simulink subsystem "TCS"  (R2025b)
settings: Solver=VariableStepAuto  StartTime=0.0  StopTime=10.0  RelTol=1e-3
settings Model: Creator=mjmag  LastModifiedBy=diego
settings RTWCC: GPUComputeCapability=3.5

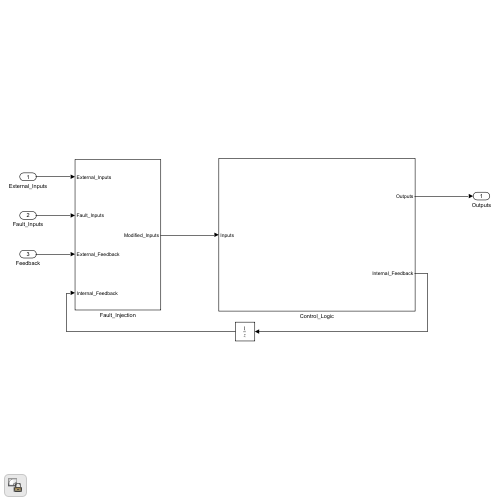
[thumbnail: Simulink's stored preview of the top-level diagram]
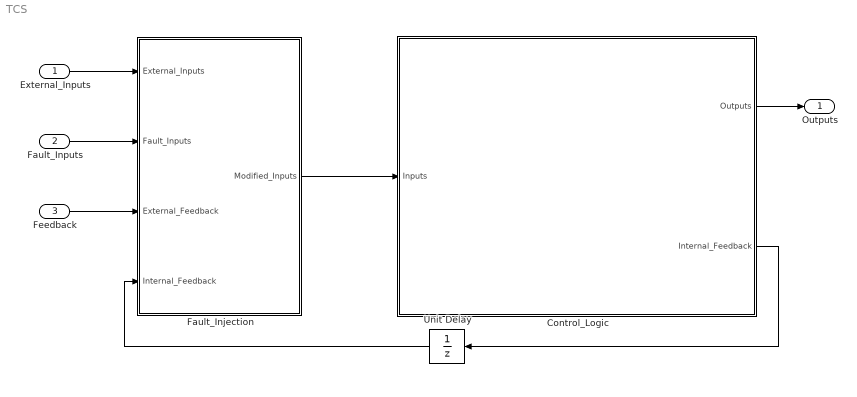
== system TCS ==
  External_Inputs : Inport
  Fault_Inputs : Inport  Port=2
  Feedback : Inport  Port=3
  Control_Logic : Subsystem
  Fault_Injection : Subsystem
  Unit Delay : UnitDelay  SampleTime=-1  HasFrameUpgradeWarning=on
  Outputs : Outport
  wires:
  Fault_Injection/1(Modified_Inputs) -> Control_Logic/1(Inputs)
  Fault_Inputs/1 -> Fault_Injection/2(Fault_Inputs)
  Control_Logic/2(Internal_Feedback) -> Unit Delay/1
  External_Inputs/1 -> Fault_Injection/1(External_Inputs)
  Feedback/1 -> Fault_Injection/3(External_Feedback)
  Unit Delay/1 -> Fault_Injection/4(Internal_Feedback)
  Control_Logic/1(Outputs) -> Outputs/1

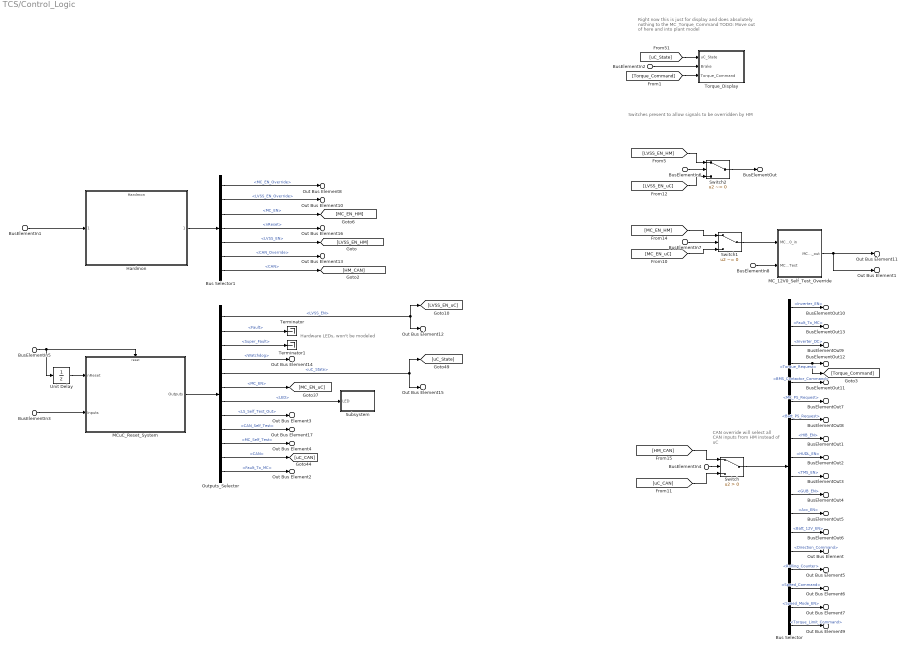
== system TCS/Control_Logic ==
  note: Right now this is just for display and does absolutely nothing to the MC_Torque_Command
      |
      | TODO: Move out of here and into plant model
  note: Switches present to allow signals
      | to be overridden by HM
  note: CAN override will select all CAN inputs from HM instead of uC
  note: Hardware LEDs, won't be modeled
  BusElementIn3 : Inport  PortName=Inputs
  BusElementIn1 : Inport  PortName=Inputs
  BusElementIn2 : Inport  PortName=Inputs  Element=Rider_Inputs.Brake
  BusElementIn4 : Inport  PortName=Inputs  Element=Feedback.Internal_Feedback.CAN_Override
  BusElementIn5 : Inport  PortName=Inputs  Element=Feedback.Internal_Feedback.nReset
  BusElementIn6 : Inport  PortName=Inputs  Element=Feedback.Internal_Feedback.LVSS_EN_Override
  BusElementIn7 : Inport  PortName=Inputs  Element=Feedback.Internal_Feedback.MC_EN_Override
  BusElementIn8 : Inport  PortName=Inputs  Element=Feedback.Internal_Feedback.MC_Self_Test
  Bus Selector : BusSelector  OutputSignals=Inverter_EN,Fault_To_MC,Inverter_DC,Torque_Request,BMS_Contactor_Command,MC_PS_Request,Batt_PS_Request,HIB_EN,HUDL_EN,TMS_EN,GUB_EN,Acc_EN,Batt_12V_EN,Direction_Command,Rolling_Counter,Speed_Command,Speed_Mode_EN,Torque_Limit_Command
  Bus Selector1 : BusSelector  OutputSignals=MC_EN_Override,LVSS_EN_Override,MC_EN,nReset,LVSS_EN,CAN_Override,CAN
  Hardmon : ModelReference  ModelNameDialog=Hardmon  SimulationMode=Normal  ModelReferenceVersion=1.106
  MC_12V0_Self_Test_Override : Subsystem
  "MCuC_Reset_System " : Subsystem  TreatAsAtomicUnit=on
  Outputs_Selector : BusSelector  OutputSignals=LVSS_EN,Fault,Super_Fault,Watchdog,uC_State,MC_EN,LED,LS_Self_Test_Out,CAN_Self_Test,MC_Self_Test,CAN,CAN.Fault_To_MC
  Subsystem : Subsystem
  Switch : Switch  Criteria=u2 > Threshold  OutDataTypeStr=Inherit: Inherit via back propagation  SaturateOnIntegerOverflow=off  InputSameDT=off
  Switch1 : Switch  Criteria=u2 ~= 0  SaturateOnIntegerOverflow=off  InputSameDT=off
  Switch2 : Switch  Criteria=u2 ~= 0  SaturateOnIntegerOverflow=off  InputSameDT=off
  Terminator : Terminator
  Terminator1 : Terminator
  Torque_Display : Subsystem
  Unit Delay : UnitDelay  SampleTime=-1  HasFrameUpgradeWarning=on
  Out Bus Element : Outport  PortName=Outputs  Element=MC_Outputs.MC_Command.Direction_Command
  Out Bus Element5 : Outport  PortName=Outputs  Element=MC_Outputs.MC_Command.Rolling_Counter
  Out Bus Element6 : Outport  PortName=Outputs  Element=MC_Outputs.MC_Command.Speed_Command
  Out Bus Element7 : Outport  PortName=Outputs  Element=MC_Outputs.MC_Command.Speed_Mode_Enable
  Out Bus Element9 : Outport  PortName=Outputs  Element=MC_Outputs.MC_Command.Torque_Limit_Command
  Out Bus Element2 : Outport  PortName=Outputs  Element=MC_Outputs.Fault_To_MC
  Out Bus Element1 : Outport  PortName=Outputs  Element=MC_Outputs.MC_12V0
  BusElementOut1 : Outport  PortName=Outputs  Element=LVSS_Outputs.HIB_EN
  BusElementOut2 : Outport  PortName=Outputs  Element=LVSS_Outputs.HUDL_EN
  BusElementOut3 : Outport  PortName=Outputs  Element=LVSS_Outputs.TMS_EN
  BusElementOut4 : Outport  PortName=Outputs  Element=LVSS_Outputs.GUB_EN
  BusElementOut5 : Outport  PortName=Outputs  Element=LVSS_Outputs.Acc_EN
  BusElementOut6 : Outport  PortName=Outputs  Element=LVSS_Outputs.Batt_12V_EN
  BusElementOut7 : Outport  PortName=Outputs  Element=TMS_Outputs.MC_Speed
  BusElementOut8 : Outport  PortName=Outputs  Element=TMS_Outputs.Batt_Speed
  BusElementOut9 : Outport  PortName=Outputs  Element=VCU_Outputs.Inverter_Discharge
  BusElementOut10 : Outport  PortName=Outputs  Element=VCU_Outputs.Inverter_Enable
  BusElementOut11 : Outport  PortName=Outputs  Element=VCU_Outputs.BMS_Contactor_Command
  BusElementOut12 : Outport  PortName=Outputs  Element=VCU_Outputs.Torque_Command
  BusElementOut13 : Outport  PortName=Outputs  Element=VCU_Outputs.Fault_To_MC
  BusElementOut : Outport  PortName=Outputs  Element=LVSS_Output.LSS_EN
  Out Bus Element12 : Outport  Port=2  PortName=Internal_Feedback  Element=LVSS_EN
  Out Bus Element14 : Outport  Port=2  PortName=Internal_Feedback  Element=Watchdog
  Out Bus Element15 : Outport  Port=2  PortName=Internal_Feedback  Element=uC_State
  Out Bus Element17 : Outport  Port=2  PortName=Internal_Feedback  Element=CAN_Self_Test
  Out Bus Element11 : Outport  Port=2  PortName=Internal_Feedback  Element=MC_12V0
  Out Bus Element3 : Outport  Port=2  PortName=Internal_Feedback  Element=LS_Self_Test
  Out Bus Element4 : Outport  Port=2  PortName=Internal_Feedback  Element=MC_Self_Test
  Out Bus Element8 : Outport  Port=2  PortName=Internal_Feedback  Element=MC_EN_Override
  Out Bus Element10 : Outport  Port=2  PortName=Internal_Feedback  Element=LVSS_EN_Override
  Out Bus Element13 : Outport  Port=2  PortName=Internal_Feedback  Element=CAN_Override
  Out Bus Element16 : Outport  Port=2  PortName=Internal_Feedback  Element=nReset
  wires:
  Bus Selector/18 -> Out Bus Element9/1  "<Torque_Limit_Command>"
  Bus Selector/17 -> Out Bus Element7/1  "<Speed_Mode_EN>"
  Bus Selector/16 -> Out Bus Element6/1  "<Speed_Command>"
  Bus Selector/15 -> Out Bus Element5/1  "<Rolling_Counter>"
  Bus Selector/14 -> Out Bus Element/1  "<Direction_Command>"
  Bus Selector/13 -> BusElementOut6/1  "<Batt_12V_EN>"
  Bus Selector/12 -> BusElementOut5/1  "<Acc_EN>"
  Bus Selector/11 -> BusElementOut4/1  "<GUB_EN>"
  Bus Selector/10 -> BusElementOut3/1  "<TMS_EN>"
  Bus Selector/9 -> BusElementOut2/1  "<HUDL_EN>"
  Bus Selector/8 -> BusElementOut1/1  "<HIB_EN>"
  Bus Selector/7 -> BusElementOut8/1  "<Batt_PS_Request>"
  Bus Selector/6 -> BusElementOut7/1  "<MC_PS_Request>"
  Bus Selector/5 -> BusElementOut11/1  "<BMS_Contactor_Command>"
  [Torque_Command] -> Torque_Display/3(Torque_Command)
  Bus Selector/4 -> BusElementOut12/1, [Torque_Command]  "<Torque_Request>"
  Bus Selector/3 -> BusElementOut9/1  "<Inverter_DC>"
  Bus Selector/2 -> BusElementOut13/1  "<Fault_To_MC>"
  Bus Selector/1 -> BusElementOut10/1  "<Inverter_EN>"
  Bus Selector1/7 -> [HM_CAN]  "<CAN>"
  Bus Selector1/6 -> Out Bus Element13/1  "<CAN_Override>"
  Bus Selector1/5 -> [LVSS_EN_HM]  "<LVSS_EN>"
  Bus Selector1/4 -> Out Bus Element16/1  "<nReset>"
  Bus Selector1/3 -> [MC_EN_HM]  "<MC_EN>"
  Bus Selector1/2 -> Out Bus Element10/1  "<LVSS_EN_Override>"
  Bus Selector1/1 -> Out Bus Element8/1  "<MC_EN_Override>"
  Hardmon/1 -> Bus Selector1/1
  BusElementIn1/1 -> Hardmon/1
  Outputs_Selector/11 -> [uC_CAN]  "<CAN>"
  Outputs_Selector/12 -> Out Bus Element2/1  "<Fault_To_MC>"
  Outputs_Selector/3 -> Terminator1/1  "<Super_Fault>"
  Outputs_Selector/2 -> Terminator/1  "<Fault>"
  Outputs_Selector/10 -> Out Bus Element4/1  "<MC_Self_Test>"
  Outputs_Selector/8 -> Out Bus Element3/1  "<LS_Self_Test_Out>"
  "MCuC_Reset_System "/1(Outputs) -> Outputs_Selector/1
  BusElementIn3/1 -> "MCuC_Reset_System "/2(Inputs)
  Outputs_Selector/5 -> [uC_State], Out Bus Element15/1  "<uC_State>"
  Outputs_Selector/4 -> Out Bus Element14/1  "<Watchdog>"
  Outputs_Selector/1 -> [LVSS_EN_uC], Out Bus Element12/1  "<LVSS_EN>"
  Outputs_Selector/7 -> Subsystem/1(LED)  "<LED>"
  Outputs_Selector/9 -> Out Bus Element17/1  "<CAN_Self_Test>"
  Outputs_Selector/6 -> [MC_EN_uC]  "<MC_EN>"
  [HM_CAN] -> Switch/1
  [LVSS_EN_HM] -> Switch2/1
  Switch2/1 -> BusElementOut/1
  BusElementIn6/1 -> Switch2/2
  [LVSS_EN_uC] -> Switch2/3
  BusElementIn8/1 -> MC_12V0_Self_Test_Override/2(MC_Self_Test)
  MC_12V0_Self_Test_Override/1(MC_12V0_out) -> Out Bus Element1/1, Out Bus Element11/1
  [MC_EN_HM] -> Switch1/1
  BusElementIn7/1 -> Switch1/2
  Switch1/1 -> MC_12V0_Self_Test_Override/1(MC_12V0_in)
  [MC_EN_uC] -> Switch1/3
  BusElementIn5/1 -> "MCuC_Reset_System "/Reset, Unit Delay/1
  Switch/1 -> Bus Selector/1
  [uC_CAN] -> Switch/3
  BusElementIn4/1 -> Switch/2
  Unit Delay/1 -> "MCuC_Reset_System "/1(nReset)
  [uC_State] -> Torque_Display/1(uC_State)
  BusElementIn2/1 -> Torque_Display/2(Brake)

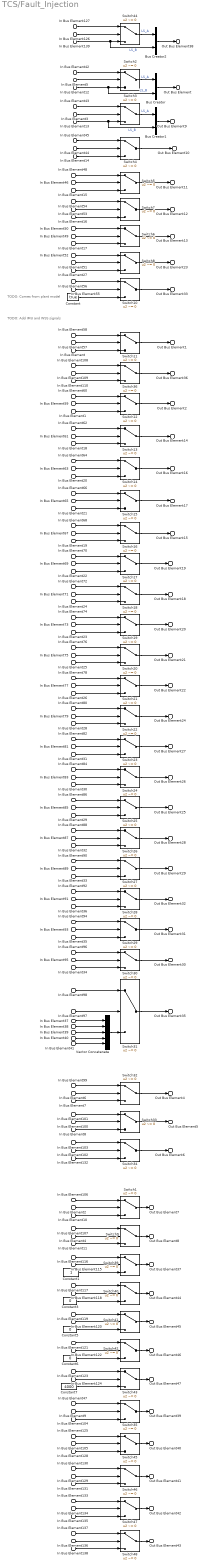
== system TCS/Fault_Injection ==
  note: TODO: Add IMU and WSS signals
  note: TODO: Comes from plant model
  In Bus Element12 : Inport  PortName=External_Inputs  Element=No_HIB.Key_In
  In Bus Element13 : Inport  PortName=External_Inputs  Element=No_HIB.Estop_In
  In Bus Element17 : Inport  PortName=External_Inputs  Element=Yes_HIB.Throttle
  In Bus Element16 : Inport  PortName=External_Inputs  Element=Yes_HIB.Start
  In Bus Element15 : Inport  PortName=External_Inputs  Element=Yes_HIB.Forward_EN
  In Bus Element14 : Inport  PortName=External_Inputs  Element=Yes_HIB.Brake
  In Bus Element27 : Inport  PortName=External_Inputs  Element=Yes_HIB.HIB_Comparison_Fault
  In Bus Element41 : Inport  PortName=External_Inputs  Element=Yes_HIB.HIB_Heartbeat
  In Bus Element2 : Inport  Port=2  PortName=Fault_Inputs  Element=Override_Watchdog
  In Bus Element3 : Inport  Port=2  PortName=Fault_Inputs  Element=Override_Back_Wheel_Speed
  In Bus Element4 : Inport  Port=2  PortName=Fault_Inputs  Element=Override_uC_State
  In Bus Element5 : Inport  Port=2  PortName=Fault_Inputs  Element=Override_Front_Wheel_Speed
  In Bus Element42 : Inport  Port=2  PortName=Fault_Inputs  Element=Front_Wheel_Speed
  In Bus Element43 : Inport  Port=2  PortName=Fault_Inputs  Element=Back_Wheel_Speed
  In Bus Element44 : Inport  Port=2  PortName=Fault_Inputs  Element=Override_Brake
  In Bus Element45 : Inport  Port=2  PortName=Fault_Inputs  Element=Brake
  In Bus Element46 : Inport  Port=2  PortName=Fault_Inputs  Element=Override_Forward_EN
  In Bus Element48 : Inport  Port=2  PortName=Fault_Inputs  Element=Forward_EN
  In Bus Element53 : Inport  Port=2  PortName=Fault_Inputs  Element=Override_Start
  In Bus Element54 : Inport  Port=2  PortName=Fault_Inputs  Element=Start
  In Bus Element50 : Inport  Port=2  PortName=Fault_Inputs  Element=Throttle
  In Bus Element49 : Inport  Port=2  PortName=Fault_Inputs  Element=Override_Throttle
  In Bus Element51 : Inport  Port=2  PortName=Fault_Inputs  Element=Override_HIB_Comparison_Fault
  In Bus Element52 : Inport  Port=2  PortName=Fault_Inputs  Element=HIB_Comparison_Fault
  In Bus Element56 : Inport  Port=2  PortName=Fault_Inputs  Element=Interlock
  In Bus Element55 : Inport  Port=2  PortName=Fault_Inputs  Element=Override_Interlock
  In Bus Element59 : Inport  Port=2  PortName=Fault_Inputs  Element=Override_LVSS_ON
  In Bus Element60 : Inport  Port=2  PortName=Fault_Inputs  Element=LVSS_ON
  In Bus Element61 : Inport  Port=2  PortName=Fault_Inputs  Element=Override_Contactor_Closed
  In Bus Element62 : Inport  Port=2  PortName=Fault_Inputs  Element=Contactor_Closed
  In Bus Element63 : Inport  Port=2  PortName=Fault_Inputs  Element=Override_Cell_Temps
  In Bus Element64 : Inport  Port=2  PortName=Fault_Inputs  Element=Cell_Temps
  In Bus Element65 : Inport  Port=2  PortName=Fault_Inputs  Element=Override_Cell_Voltages
  In Bus Element66 : Inport  Port=2  PortName=Fault_Inputs  Element=Cell_Voltages
  In Bus Element67 : Inport  Port=2  PortName=Fault_Inputs  Element=Override_Isolation_State
  In Bus Element68 : Inport  Port=2  PortName=Fault_Inputs  Element=Isolation_State
  In Bus Element69 : Inport  Port=2  PortName=Fault_Inputs  Element=Override_MC_Speed_Out
  In Bus Element70 : Inport  Port=2  PortName=Fault_Inputs  Element=MC_Speed_Out
  In Bus Element71 : Inport  Port=2  PortName=Fault_Inputs  Element=Override_Batt_Speed_Out
  In Bus Element72 : Inport  Port=2  PortName=Fault_Inputs  Element=Batt_Speed_Out
  In Bus Element73 : Inport  Port=2  PortName=Fault_Inputs  Element=Override_Temperatures
  In Bus Element74 : Inport  Port=2  PortName=Fault_Inputs  Element=Temperatures
  In Bus Element75 : Inport  Port=2  PortName=Fault_Inputs  Element=Override_MC_Flow_Rate
  In Bus Element76 : Inport  Port=2  PortName=Fault_Inputs  Element=MC_Flow_Rate
  In Bus Element77 : Inport  Port=2  PortName=Fault_Inputs  Element=Override_Batt_Flow_Rate
  In Bus Element78 : Inport  Port=2  PortName=Fault_Inputs  Element=Batt_Flow_Rate
  In Bus Element79 : Inport  Port=2  PortName=Fault_Inputs  Element=Override_HIB_ON
  In Bus Element80 : Inport  Port=2  PortName=Fault_Inputs  Element=HIB_ON
  In Bus Element81 : Inport  Port=2  PortName=Fault_Inputs  Element=Override_HUDL_ON
  In Bus Element82 : Inport  Port=2  PortName=Fault_Inputs  Element=HUDL_ON
  In Bus Element83 : Inport  Port=2  PortName=Fault_Inputs  Element=Override_TMS_ON
  In Bus Element84 : Inport  Port=2  PortName=Fault_Inputs  Element=TMS_ON
  In Bus Element85 : Inport  Port=2  PortName=Fault_Inputs  Element=Override_GUB_ON
  In Bus Element86 : Inport  Port=2  PortName=Fault_Inputs  Element=GUB_ON
  In Bus Element87 : Inport  Port=2  PortName=Fault_Inputs  Element=Override_Acc_ON
  In Bus Element88 : Inport  Port=2  PortName=Fault_Inputs  Element=Acc_ON
  In Bus Element89 : Inport  Port=2  PortName=Fault_Inputs  Element=Override_Batt_12V_ON
  In Bus Element90 : Inport  Port=2  PortName=Fault_Inputs  Element=Batt_12V_ON
  In Bus Element91 : Inport  Port=2  PortName=Fault_Inputs  Element=Override_Vicor_Current
  In Bus Element92 : Inport  Port=2  PortName=Fault_Inputs  Element=Vicor_Current
  In Bus Element93 : Inport  Port=2  PortName=Fault_Inputs  Element=Override_LVSS_Temps
  In Bus Element94 : Inport  Port=2  PortName=Fault_Inputs  Element=LVSS_Temps
  In Bus Element95 : Inport  Port=2  PortName=Fault_Inputs  Element=Override_LVSS_Currents
  In Bus Element96 : Inport  Port=2  PortName=Fault_Inputs  Element=LVSS_Currents
  In Bus Element97 : Inport  Port=2  PortName=Fault_Inputs  Element=Override_Heartbeats
  In Bus Element98 : Inport  Port=2  PortName=Fault_Inputs  Element=Heartbeats
  In Bus Element6 : Inport  Port=2  PortName=Fault_Inputs  Element=Override_MC_12V0
  In Bus Element99 : Inport  Port=2  PortName=Fault_Inputs  Element=MC_12V0
  In Bus Element100 : Inport  Port=2  PortName=Fault_Inputs  Element=Override_LVSS_EN
  In Bus Element101 : Inport  Port=2  PortName=Fault_Inputs  Element=LVSS_EN
  In Bus Element102 : Inport  Port=2  PortName=Fault_Inputs  Element=Override_nReset
  In Bus Element103 : Inport  Port=2  PortName=Fault_Inputs  Element=nReset
  In Bus Element106 : Inport  Port=2  PortName=Fault_Inputs  Element=Watchdog
  In Bus Element107 : Inport  Port=2  PortName=Fault_Inputs  Element=uC_State
  In Bus Element57 : Inport  Port=2  PortName=Fault_Inputs  Element=Override_Inverter_Discharge_State
  In Bus Element58 : Inport  Port=2  PortName=Fault_Inputs  Element=Inverter_Discharge_State
  In Bus Element109 : Inport  Port=2  PortName=Fault_Inputs  Element=Override_VSM_State
  In Bus Element108 : Inport  Port=2  PortName=Fault_Inputs  Element=VSM_State
  In Bus Element116 : Inport  Port=2  PortName=Fault_Inputs  Element=Direction_Command
  In Bus Element115 : Inport  Port=2  PortName=Fault_Inputs  Element=Override_Direction_Command
  In Bus Element117 : Inport  Port=2  PortName=Fault_Inputs  Element=Rolling_Counter
  In Bus Element118 : Inport  Port=2  PortName=Fault_Inputs  Element=Override_Rolling_Counter
  In Bus Element119 : Inport  Port=2  PortName=Fault_Inputs  Element=Speed_Command
  In Bus Element120 : Inport  Port=2  PortName=Fault_Inputs  Element=Override_Speed_Command
  In Bus Element121 : Inport  Port=2  PortName=Fault_Inputs  Element=Speed_Mode_Enable
  In Bus Element122 : Inport  Port=2  PortName=Fault_Inputs  Element=Override_Speed_Mode_Enable
  In Bus Element123 : Inport  Port=2  PortName=Fault_Inputs  Element=Torque_Limit_Command
  In Bus Element124 : Inport  Port=2  PortName=Fault_Inputs  Element=Override_Torque_Limit_Command
  In Bus Element127 : Inport  Port=2  PortName=Fault_Inputs  Element=LS_Self_Test
  In Bus Element126 : Inport  Port=2  PortName=Fault_Inputs  Element=Override_LS_Self_Test
  In Bus Element9 : Inport  Port=2  PortName=Fault_Inputs  Element=Override_CAN_Override
  In Bus Element47 : Inport  Port=2  PortName=Fault_Inputs  Element=CAN_Override
  In Bus Element125 : Inport  Port=2  PortName=Fault_Inputs  Element=LVSS_EN_Override
  In Bus Element105 : Inport  Port=2  PortName=Fault_Inputs  Element=Override_LVSS_EN_Override
  In Bus Element130 : Inport  Port=2  PortName=Fault_Inputs  Element=MC_EN_Override
  In Bus Element129 : Inport  Port=2  PortName=Fault_Inputs  Element=Override_MC_EN_Override
  In Bus Element133 : Inport  Port=2  PortName=Fault_Inputs  Element=MC_Self_Test
  In Bus Element134 : Inport  Port=2  PortName=Fault_Inputs  Element=Override_MC_Self_Test
  In Bus Element137 : Inport  Port=2  PortName=Fault_Inputs  Element=CAN_Self_Test
  In Bus Element136 : Inport  Port=2  PortName=Fault_Inputs  Element=Override_CAN_Self_Test
  In Bus Element : Inport  Port=3  PortName=External_Feedback  Element=MC_Feedback.D4_Inverter_Discharge_State
  In Bus Element110 : Inport  Port=3  PortName=External_Feedback  Element=MC_Feedback.D1_VSM_State
  In Bus Element28 : Inport  Port=3  PortName=External_Feedback  Element=LVSS_Feedback.HIB_ON
  In Bus Element1 : Inport  Port=3  PortName=External_Feedback  Element=LVSS_Feedback.LVSS_ON
  In Bus Element31 : Inport  Port=3  PortName=External_Feedback  Element=LVSS_Feedback.HUDL_ON
  In Bus Element30 : Inport  Port=3  PortName=External_Feedback  Element=LVSS_Feedback.TMS_ON
  In Bus Element29 : Inport  Port=3  PortName=External_Feedback  Element=LVSS_Feedback.GUB_ON
  In Bus Element32 : Inport  Port=3  PortName=External_Feedback  Element=LVSS_Feedback.Acc_ON
  In Bus Element33 : Inport  Port=3  PortName=External_Feedback  Element=LVSS_Feedback.Batt_12V_ON
  In Bus Element36 : Inport  Port=3  PortName=External_Feedback  Element=LVSS_Feedback.Vicor_Current
  In Bus Element35 : Inport  Port=3  PortName=External_Feedback  Element=LVSS_Feedback.LVSS_Temps
  In Bus Element34 : Inport  Port=3  PortName=External_Feedback  Element=LVSS_Feedback.LVSS_Currents
  In Bus Element37 : Inport  Port=3  PortName=External_Feedback  Element=LVSS_Feedback.LVSS_Heartbeat
  In Bus Element18 : Inport  Port=3  PortName=External_Feedback  Element=BMS_Feedback.BMS_Feedback.Contactor_Closed
  In Bus Element20 : Inport  Port=3  PortName=External_Feedback  Element=BMS_Feedback.BMS_Feedback.Cell_Temps
  In Bus Element21 : Inport  Port=3  PortName=External_Feedback  Element=BMS_Feedback.BMS_Feedback.Cell_Voltages
  In Bus Element39 : Inport  Port=3  PortName=External_Feedback  Element=BMS_Feedback.BMS_Feedback.BMS_Heartbeat
  In Bus Element19 : Inport  Port=3  PortName=External_Feedback  Element=GFDB_Feedback.GFDB_Feedback.Isolation_State
  In Bus Element40 : Inport  Port=3  PortName=External_Feedback  Element=GFDB_Feedback.GFDB_Feedback.GFDB_Heartbeat
  In Bus Element22 : Inport  Port=3  PortName=External_Feedback  Element=TMS_Feedback.MC_Speed_Out
  In Bus Element24 : Inport  Port=3  PortName=External_Feedback  Element=TMS_Feedback.Batt_Speed_Out
  In Bus Element23 : Inport  Port=3  PortName=External_Feedback  Element=TMS_Feedback.Temperatures
  In Bus Element25 : Inport  Port=3  PortName=External_Feedback  Element=TMS_Feedback.MC_Flow_Rate
  In Bus Element26 : Inport  Port=3  PortName=External_Feedback  Element=TMS_Feedback.Batt_Flow_Rate
  In Bus Element38 : Inport  Port=3  PortName=External_Feedback  Element=TMS_Feedback.TMS_Heartbeat
  In Bus Element7 : Inport  Port=4  PortName=Internal_Feedback  Element=MC_12V0
  In Bus Element8 : Inport  Port=4  PortName=Internal_Feedback  Element=LVSS_EN
  In Bus Element10 : Inport  Port=4  PortName=Internal_Feedback  Element=Watchdog
  In Bus Element11 : Inport  Port=4  PortName=Internal_Feedback  Element=uC_State
  In Bus Element104 : Inport  Port=4  PortName=Internal_Feedback  Element=CAN_Override
  In Bus Element128 : Inport  Port=4  PortName=Internal_Feedback  Element=LVSS_EN_Override
  In Bus Element131 : Inport  Port=4  PortName=Internal_Feedback  Element=MC_EN_Override
  In Bus Element132 : Inport  Port=4  PortName=Internal_Feedback  Element=nReset
  In Bus Element135 : Inport  Port=4  PortName=Internal_Feedback  Element=MC_Self_Test
  In Bus Element138 : Inport  Port=4  PortName=Internal_Feedback  Element=CAN_Self_Test
  In Bus Element139 : Inport  Port=4  PortName=Internal_Feedback  Element=LS_Self_Test
  Bus Creator : BusCreator  Inputs=2
  Bus Creator1 : BusCreator  Inputs=2
  Bus Creator2 : BusCreator  Inputs=2
  Constant : Constant  Value=true
  Constant1 : Constant
  Constant3 : Constant  Value=0
  Constant5 : Constant  Value=0
  Constant6 : Constant  Value=0
  Constant7 : Constant  Value=4000
  Switch{1..36,39..48} (46 alike) : Switch  Criteria=u2 ~= 0  OutDataTypeStr=Inherit: Inherit via back propagation  SaturateOnIntegerOverflow=off  InputSameDT=off
  Vector Concatenate : Concatenate  NumInputs=5
  Out Bus Element : Outport  PortName=Modified_Inputs  Element=Rider_Inputs.Key_In
  Out Bus Element9 : Outport  PortName=Modified_Inputs  Element=Rider_Inputs.Estop_In
  Out Bus Element10 : Outport  PortName=Modified_Inputs  Element=Rider_Inputs.Brake
  Out Bus Element11 : Outport  PortName=Modified_Inputs  Element=Rider_Inputs.Forward_EN
  Out Bus Element12 : Outport  PortName=Modified_Inputs  Element=Rider_Inputs.Start
  Out Bus Element13 : Outport  PortName=Modified_Inputs  Element=Rider_Inputs.Throttle
  Out Bus Element1 : Outport  PortName=Modified_Inputs  Element=Feedback.MC_Feedback.D4_Inverter_Discharge_State
  Out Bus Element36 : Outport  PortName=Modified_Inputs  Element=Feedback.MC_Feedback.D1_VSM_State
  Out Bus Element2 : Outport  PortName=Modified_Inputs  Element=Feedback.LVSS_Feedback.LVSS_ON
  Out Bus Element24 : Outport  PortName=Modified_Inputs  Element=Feedback.LVSS_Feedback.HIB_ON
  Out Bus Element25 : Outport  PortName=Modified_Inputs  Element=Feedback.LVSS_Feedback.GUB_ON
  Out Bus Element26 : Outport  PortName=Modified_Inputs  Element=Feedback.LVSS_Feedback.TMS_ON
  Out Bus Element27 : Outport  PortName=Modified_Inputs  Element=Feedback.LVSS_Feedback.HUDL_ON
  Out Bus Element28 : Outport  PortName=Modified_Inputs  Element=Feedback.LVSS_Feedback.Acc_ON
  Out Bus Element29 : Outport  PortName=Modified_Inputs  Element=Feedback.LVSS_Feedback.Batt_12V_ON
  Out Bus Element30 : Outport  PortName=Modified_Inputs  Element=Feedback.LVSS_Feedback.LVSS_Currents
  Out Bus Element31 : Outport  PortName=Modified_Inputs  Element=Feedback.LVSS_Feedback.LVSS_Temps
  Out Bus Element32 : Outport  PortName=Modified_Inputs  Element=Feedback.LVSS_Feedback.Vicor_Current
  Out Bus Element4 : Outport  PortName=Modified_Inputs  Element=Feedback.Internal_Feedback.MC_12V0
  Out Bus Element5 : Outport  PortName=Modified_Inputs  Element=Feedback.Internal_Feedback.LVSS_EN_uC
  Out Bus Element6 : Outport  PortName=Modified_Inputs  Element=Feedback.Internal_Feedback.nReset
  Out Bus Element7 : Outport  PortName=Modified_Inputs  Element=Feedback.Internal_Feedback.Watchdog
  Out Bus Element8 : Outport  PortName=Modified_Inputs  Element=Feedback.Internal_Feedback.uC_State
  Out Bus Element39 : Outport  PortName=Modified_Inputs  Element=Feedback.Internal_Feedback.CAN_Override
  Out Bus Element40 : Outport  PortName=Modified_Inputs  Element=Feedback.Internal_Feedback.LVSS_EN_Override
  Out Bus Element41 : Outport  PortName=Modified_Inputs  Element=Feedback.Internal_Feedback.MC_EN_Override
  Out Bus Element42 : Outport  PortName=Modified_Inputs  Element=Feedback.Internal_Feedback.MC_Self_Test
  Out Bus Element43 : Outport  PortName=Modified_Inputs  Element=Feedback.Internal_Feedback.CAN_Self_Test
  Out Bus Element14 : Outport  PortName=Modified_Inputs  Element=Feedback.BMS_Feedback.Contactor_Closed
  Out Bus Element16 : Outport  PortName=Modified_Inputs  Element=Feedback.BMS_Feedback.Cell_Temps
  Out Bus Element17 : Outport  PortName=Modified_Inputs  Element=Feedback.BMS_Feedback.Cell_Voltages
  Out Bus Element15 : Outport  PortName=Modified_Inputs  Element=Feedback.GFDB_Feedback.Isolation_State
  Out Bus Element19 : Outport  PortName=Modified_Inputs  Element=Feedback.TMS_Feedback.MC_Speed_Out
  Out Bus Element18 : Outport  PortName=Modified_Inputs  Element=Feedback.TMS_Feedback.Batt_Speed_Out
  Out Bus Element20 : Outport  PortName=Modified_Inputs  Element=Feedback.TMS_Feedback.Temperatures
  Out Bus Element21 : Outport  PortName=Modified_Inputs  Element=Feedback.TMS_Feedback.MC_Flow_Rate
  Out Bus Element22 : Outport  PortName=Modified_Inputs  Element=Feedback.TMS_Feedback.Batt_Flow_Rate
  Out Bus Element35 : Outport  PortName=Modified_Inputs  Element=Feedback.Heartbeats
  Out Bus Element23 : Outport  PortName=Modified_Inputs  Element=HIB.HIB_Comparison_Fault
  Out Bus Element33 : Outport  PortName=Modified_Inputs  Element=Interlock
  Out Bus Element37 : Outport  PortName=Modified_Inputs  Element=MC_Direction_Command
  Out Bus Element44 : Outport  PortName=Modified_Inputs  Element=MC_Rolling_Counter
  Out Bus Element45 : Outport  PortName=Modified_Inputs  Element=MC_Speed_Command
  Out Bus Element46 : Outport  PortName=Modified_Inputs  Element=MC_Speed_Mode_Enable
  Out Bus Element47 : Outport  PortName=Modified_Inputs  Element=MC_Torque_Limit_Command
  Out Bus Element38 : Outport  PortName=Modified_Inputs  Element=Internal_Feedback.LS_Self_Test
  wires:
  In Bus Element138/1 -> Switch48/3
  In Bus Element136/1 -> Switch48/2
  In Bus Element137/1 -> Switch48/1
  Switch48/1 -> Out Bus Element43/1
  Switch47/1 -> Out Bus Element42/1
  In Bus Element133/1 -> Switch47/1
  In Bus Element134/1 -> Switch47/2
  In Bus Element135/1 -> Switch47/3
  In Bus Element131/1 -> Switch46/3
  In Bus Element129/1 -> Switch46/2
  In Bus Element130/1 -> Switch46/1
  Switch46/1 -> Out Bus Element41/1
  Switch45/1 -> Out Bus Element40/1
  In Bus Element125/1 -> Switch45/1
  In Bus Element105/1 -> Switch45/2
  In Bus Element128/1 -> Switch45/3
  In Bus Element104/1 -> Switch35/3
  In Bus Element9/1 -> Switch35/2
  In Bus Element47/1 -> Switch35/1
  Switch35/1 -> Out Bus Element39/1
  In Bus Element132/1 -> Switch34/3
  In Bus Element139/1 -> Switch44/3, Bus Creator2/2  "LS_B"
  In Bus Element126/1 -> Switch44/2
  Switch44/1 -> Bus Creator2/1  "LS_A"
  Bus Creator2/1 -> Out Bus Element38/1
  In Bus Element127/1 -> Switch44/1
  Constant7/1 -> Switch43/3
  Constant6/1 -> Switch42/3
  Constant5/1 -> Switch41/3
  Constant3/1 -> Switch40/3
  Constant1/1 -> Switch39/3
  In Bus Element124/1 -> Switch43/2
  In Bus Element123/1 -> Switch43/1
  In Bus Element122/1 -> Switch42/2
  In Bus Element121/1 -> Switch42/1
  In Bus Element120/1 -> Switch41/2
  In Bus Element119/1 -> Switch41/1
  In Bus Element118/1 -> Switch40/2
  In Bus Element117/1 -> Switch40/1
  In Bus Element115/1 -> Switch39/2
  In Bus Element116/1 -> Switch39/1
  Switch43/1 -> Out Bus Element47/1
  Switch42/1 -> Out Bus Element46/1
  Switch41/1 -> Out Bus Element45/1
  Switch40/1 -> Out Bus Element44/1
  Switch39/1 -> Out Bus Element37/1
  In Bus Element108/1 -> Switch36/1
  In Bus Element110/1 -> Switch36/3
  Switch36/1 -> Out Bus Element36/1
  In Bus Element109/1 -> Switch36/2
  In Bus Element41/1 -> Vector Concatenate/5
  In Bus Element40/1 -> Vector Concatenate/4
  In Bus Element37/1 -> Vector Concatenate/1
  In Bus Element38/1 -> Vector Concatenate/2
  In Bus Element39/1 -> Vector Concatenate/3
  In Bus Element13/1 -> Switch3/3, Bus Creator1/2  "LS_B"
  Bus Creator1/1 -> Out Bus Element9/1
  In Bus Element43/1 -> Switch3/1
  Switch3/1 -> Bus Creator1/1  "LS_A"
  In Bus Element3/1 -> Switch3/2
  In Bus Element5/1 -> Switch2/2
  Switch2/1 -> Bus Creator/1  "LS_A"
  In Bus Element42/1 -> Switch2/1
  Bus Creator/1 -> Out Bus Element/1
  In Bus Element12/1 -> Switch2/3, Bus Creator/2  "LS_B"
  In Bus Element2/1 -> Switch1/2
  Switch1/1 -> Out Bus Element7/1
  In Bus Element106/1 -> Switch1/1
  Switch9/1 -> Out Bus Element8/1
  In Bus Element107/1 -> Switch9/1
  In Bus Element4/1 -> Switch9/2
  In Bus Element11/1 -> Switch9/3
  In Bus Element10/1 -> Switch1/3
  In Bus Element44/1 -> Switch4/2
  In Bus Element45/1 -> Switch4/1
  In Bus Element14/1 -> Switch4/3
  Switch4/1 -> Out Bus Element10/1
  Switch5/1 -> Out Bus Element11/1
  In Bus Element15/1 -> Switch5/3
  In Bus Element46/1 -> Switch5/2
  In Bus Element48/1 -> Switch5/1
  Switch7/1 -> Out Bus Element12/1
  In Bus Element53/1 -> Switch7/2
  In Bus Element54/1 -> Switch7/1
  In Bus Element16/1 -> Switch7/3
  In Bus Element49/1 -> Switch6/2
  In Bus Element50/1 -> Switch6/1
  Switch6/1 -> Out Bus Element13/1
  In Bus Element17/1 -> Switch6/3
  In Bus Element51/1 -> Switch8/2
  In Bus Element52/1 -> Switch8/1
  Switch8/1 -> Out Bus Element23/1
  In Bus Element27/1 -> Switch8/3
  In Bus Element55/1 -> Switch10/2
  In Bus Element56/1 -> Switch10/1
  Switch10/1 -> Out Bus Element33/1
  Constant/1 -> Switch10/3
  In Bus Element57/1 -> Switch11/2
  In Bus Element58/1 -> Switch11/1
  Switch11/1 -> Out Bus Element1/1
  In Bus Element/1 -> Switch11/3
  In Bus Element59/1 -> Switch12/2
  In Bus Element60/1 -> Switch12/1
  Switch12/1 -> Out Bus Element2/1
  In Bus Element1/1 -> Switch12/3
  In Bus Element61/1 -> Switch13/2
  In Bus Element62/1 -> Switch13/1
  Switch13/1 -> Out Bus Element14/1
  In Bus Element18/1 -> Switch13/3
  In Bus Element63/1 -> Switch14/2
  In Bus Element64/1 -> Switch14/1
  Switch14/1 -> Out Bus Element16/1
  In Bus Element20/1 -> Switch14/3
  In Bus Element65/1 -> Switch15/2
  In Bus Element66/1 -> Switch15/1
  Switch15/1 -> Out Bus Element17/1
  In Bus Element21/1 -> Switch15/3
  In Bus Element67/1 -> Switch16/2
  In Bus Element68/1 -> Switch16/1
  Switch16/1 -> Out Bus Element15/1
  In Bus Element19/1 -> Switch16/3
  In Bus Element69/1 -> Switch17/2
  In Bus Element70/1 -> Switch17/1
  Switch17/1 -> Out Bus Element19/1
  In Bus Element22/1 -> Switch17/3
  In Bus Element71/1 -> Switch18/2
  In Bus Element72/1 -> Switch18/1
  Switch18/1 -> Out Bus Element18/1
  In Bus Element24/1 -> Switch18/3
  In Bus Element73/1 -> Switch19/2
  In Bus Element74/1 -> Switch19/1
  Switch19/1 -> Out Bus Element20/1
  In Bus Element23/1 -> Switch19/3
  In Bus Element75/1 -> Switch20/2
  In Bus Element76/1 -> Switch20/1
  Switch20/1 -> Out Bus Element21/1
  In Bus Element25/1 -> Switch20/3
  In Bus Element77/1 -> Switch21/2
  In Bus Element78/1 -> Switch21/1
  Switch21/1 -> Out Bus Element22/1
  In Bus Element26/1 -> Switch21/3
  In Bus Element79/1 -> Switch22/2
  In Bus Element80/1 -> Switch22/1
  Switch22/1 -> Out Bus Element24/1
  In Bus Element28/1 -> Switch22/3
  In Bus Element81/1 -> Switch23/2
  In Bus Element82/1 -> Switch23/1
  Switch23/1 -> Out Bus Element27/1
  In Bus Element31/1 -> Switch23/3
  In Bus Element83/1 -> Switch24/2
  In Bus Element84/1 -> Switch24/1
  Switch24/1 -> Out Bus Element26/1
  In Bus Element30/1 -> Switch24/3
  In Bus Element85/1 -> Switch25/2
  In Bus Element86/1 -> Switch25/1
  Switch25/1 -> Out Bus Element25/1
  In Bus Element29/1 -> Switch25/3
  In Bus Element87/1 -> Switch26/2
  In Bus Element88/1 -> Switch26/1
  Switch26/1 -> Out Bus Element28/1
  In Bus Element32/1 -> Switch26/3
  In Bus Element89/1 -> Switch27/2
  In Bus Element90/1 -> Switch27/1
  Switch27/1 -> Out Bus Element29/1
  In Bus Element33/1 -> Switch27/3
  In Bus Element91/1 -> Switch28/2
  In Bus Element92/1 -> Switch28/1
  Switch28/1 -> Out Bus Element32/1
  In Bus Element36/1 -> Switch28/3
  In Bus Element93/1 -> Switch29/2
  In Bus Element94/1 -> Switch29/1
  Switch29/1 -> Out Bus Element31/1
  In Bus Element35/1 -> Switch29/3
  In Bus Element95/1 -> Switch30/2
  In Bus Element96/1 -> Switch30/1
  Switch30/1 -> Out Bus Element30/1
  In Bus Element34/1 -> Switch30/3
  In Bus Element97/1 -> Switch31/2
  In Bus Element98/1 -> Switch31/1
  Switch31/1 -> Out Bus Element35/1
  Vector Concatenate/1 -> Switch31/3
  In Bus Element6/1 -> Switch32/2
  In Bus Element7/1 -> Switch32/3
  In Bus Element99/1 -> Switch32/1
  Switch32/1 -> Out Bus Element4/1
  In Bus Element100/1 -> Switch33/2
  In Bus Element8/1 -> Switch33/3
  In Bus Element101/1 -> Switch33/1
  Switch33/1 -> Out Bus Element5/1
  In Bus Element102/1 -> Switch34/2
  In Bus Element103/1 -> Switch34/1
  Switch34/1 -> Out Bus Element6/1

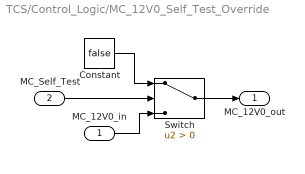
== system TCS/Control_Logic/MC_12V0_Self_Test_Override ==
  MC_12V0_in : Inport
  MC_Self_Test : Inport  Port=2
  Constant : Constant  Value=false
  Switch : Switch  Criteria=u2 > Threshold  SaturateOnIntegerOverflow=off  InputSameDT=off
  MC_12V0_out : Outport
  wires:
  MC_12V0_in/1 -> Switch/3
  Constant/1 -> Switch/1
  Switch/1 -> MC_12V0_out/1
  MC_Self_Test/1 -> Switch/2

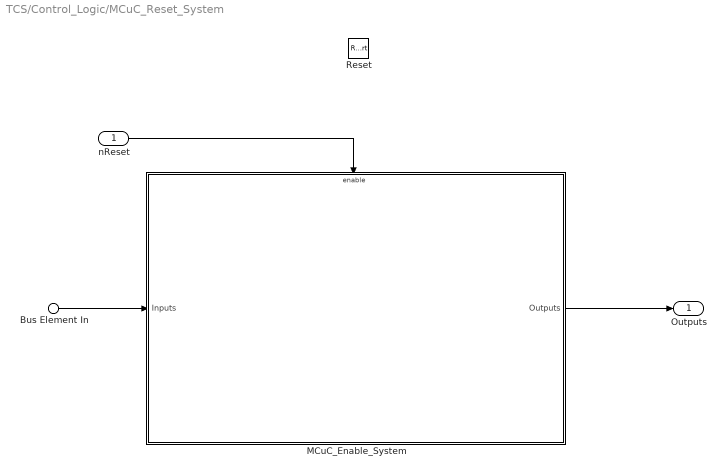
== system TCS/Control_Logic/MCuC_Reset_System  ==
  nReset : Inport
  Bus Element In : Inport  Port=2  PortName=Inputs
  Reset : ResetPort  DisableCoverage=on
  "MCuC_Enable_System " : Subsystem  TreatAsAtomicUnit=on
  Outputs : Outport
  wires:
  "MCuC_Enable_System "/1(Outputs) -> Outputs/1
  Bus Element In/1 -> "MCuC_Enable_System "/1(Inputs)
  nReset/1 -> "MCuC_Enable_System "/Enable

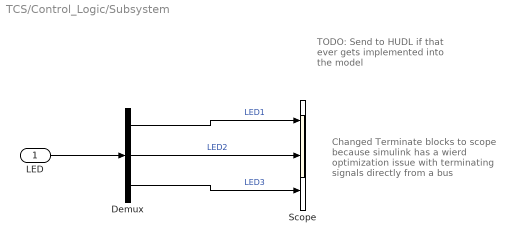
== system TCS/Control_Logic/Subsystem ==
  note: Changed Terminate blocks to scope because simulink has a wierd optimization issue with terminating signals directly from a bus
  note: TODO: Send to HUDL if that ever gets implemented into the model
  LED : Inport  PortDimensions=[1 3]
  Demux : Demux  Outputs=3
  Scope : Scope  NumInputPorts=3
  wires:
  Demux/3 -> Scope/3  "LED3"
  Demux/1 -> Scope/1  "LED1"
  Demux/2 -> Scope/2  "LED2"
  LED/1 -> Demux/1

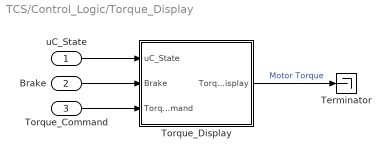
== system TCS/Control_Logic/Torque_Display ==
  uC_State : Inport
  Brake : Inport  Port=2
  Torque_Command : Inport  Port=3
  Terminator : Terminator
  Torque_Display : Stateflow chart  TreatAsAtomicUnit=on
  wires:
  Torque_Display/1(Torque_Display) -> Terminator/1  "Motor Torque"
  Brake/1 -> Torque_Display/2(Brake)
  Torque_Command/1 -> Torque_Display/3(Torque_Command)
  uC_State/1 -> Torque_Display/1(uC_State)

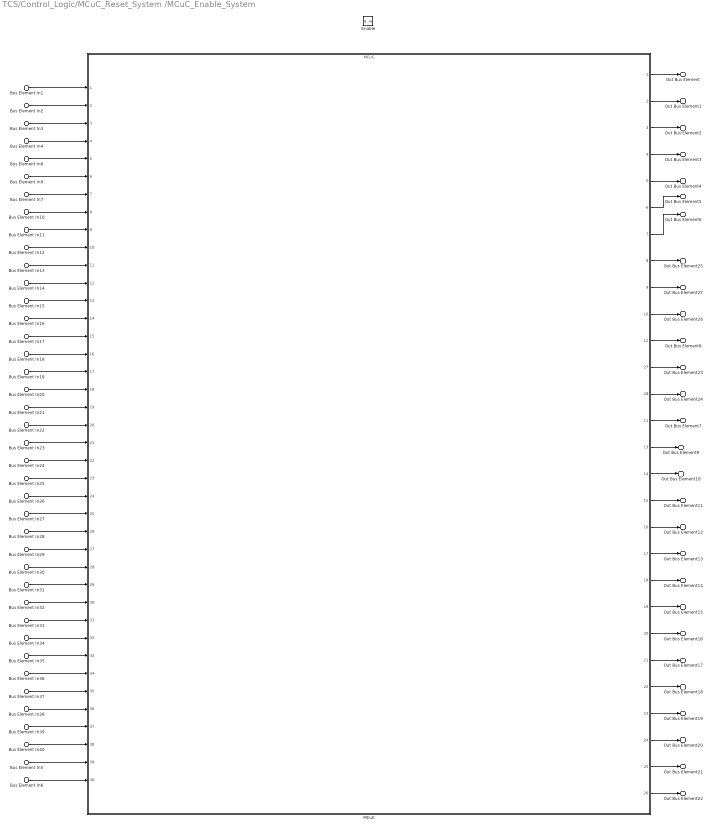
== system TCS/Control_Logic/MCuC_Reset_System /MCuC_Enable_System  ==
  Bus Element In1 : Inport  PortName=Inputs  Element=Rider_Inputs.Key_In.LS_A
  Bus Element In2 : Inport  PortName=Inputs  Element=Rider_Inputs.Key_In.LS_B
  Bus Element In3 : Inport  PortName=Inputs  Element=Rider_Inputs.Estop_In.LS_A
  Bus Element In4 : Inport  PortName=Inputs  Element=Rider_Inputs.Estop_In.LS_B
  Bus Element In9 : Inport  PortName=Inputs  Element=Rider_Inputs.Start
  Bus Element In11 : Inport  PortName=Inputs  Element=Rider_Inputs.Brake
  Bus Element In12 : Inport  PortName=Inputs  Element=Rider_Inputs.Forward_EN
  Bus Element In15 : Inport  PortName=Inputs  Element=Rider_Inputs.Throttle
  Bus Element In5 : Inport  PortName=Inputs  Element=Internal_Feedback.LS_Self_Test.LS_A
  Bus Element In6 : Inport  PortName=Inputs  Element=Internal_Feedback.LS_Self_Test.LS_B
  Bus Element In7 : Inport  PortName=Inputs  Element=Interlock
  Bus Element In8 : Inport  PortName=Inputs  Element=Feedback.Internal_Feedback.MC_12V0
  Bus Element In10 : Inport  PortName=Inputs  Element=Feedback.LVSS_Feedback.LVSS_ON
  Bus Element In26 : Inport  PortName=Inputs  Element=Feedback.LVSS_Feedback.HIB_ON
  Bus Element In27 : Inport  PortName=Inputs  Element=Feedback.LVSS_Feedback.HUDL_ON
  Bus Element In28 : Inport  PortName=Inputs  Element=Feedback.LVSS_Feedback.TMS_ON
  Bus Element In29 : Inport  PortName=Inputs  Element=Feedback.LVSS_Feedback.GUB_ON
  Bus Element In30 : Inport  PortName=Inputs  Element=Feedback.LVSS_Feedback.Acc_ON
  Bus Element In31 : Inport  PortName=Inputs  Element=Feedback.LVSS_Feedback.Batt_12V_ON
  Bus Element In32 : Inport  PortName=Inputs  Element=Feedback.LVSS_Feedback.Vicor_Current
  Bus Element In33 : Inport  PortName=Inputs  Element=Feedback.LVSS_Feedback.LVSS_Temps
  Bus Element In34 : Inport  PortName=Inputs  Element=Feedback.LVSS_Feedback.LVSS_Currents
  Bus Element In13 : Inport  PortName=Inputs  Element=Feedback.MC_Feedback.D1_VSM_State
  Bus Element In14 : Inport  PortName=Inputs  Element=Feedback.MC_Feedback.D4_Inverter_Discharge_State
  Bus Element In16 : Inport  PortName=Inputs  Element=Feedback.BMS_Feedback.Contactor_Closed
  Bus Element In17 : Inport  PortName=Inputs  Element=Feedback.BMS_Feedback.Cell_Temps
  Bus Element In18 : Inport  PortName=Inputs  Element=Feedback.BMS_Feedback.Cell_Voltages
  Bus Element In19 : Inport  PortName=Inputs  Element=Feedback.GFDB_Feedback.Isolation_State
  Bus Element In20 : Inport  PortName=Inputs  Element=Feedback.TMS_Feedback.MC_Speed_Out
  Bus Element In21 : Inport  PortName=Inputs  Element=Feedback.TMS_Feedback.Batt_Speed_Out
  Bus Element In22 : Inport  PortName=Inputs  Element=Feedback.TMS_Feedback.Temperatures
  Bus Element In23 : Inport  PortName=Inputs  Element=Feedback.TMS_Feedback.MC_Flow_Rate
  Bus Element In24 : Inport  PortName=Inputs  Element=Feedback.TMS_Feedback.Batt_Flow_Rate
  Bus Element In35 : Inport  PortName=Inputs  Element=Feedback.Heartbeats
  Bus Element In25 : Inport  PortName=Inputs  Element=HIB.HIB_Comparison_Fault
  Bus Element In36 : Inport  PortName=Inputs  Element=MC_Direction_Command
  Bus Element In37 : Inport  PortName=Inputs  Element=MC_Rolling_Counter
  Bus Element In38 : Inport  PortName=Inputs  Element=MC_Speed_Command
  Bus Element In39 : Inport  PortName=Inputs  Element=MC_Speed_Mode_Enable
  Bus Element In40 : Inport  PortName=Inputs  Element=MC_Torque_Limit_Command
  Enable : EnablePort
  MCuC : ModelReference  ModelNameDialog=MCuC.slx  SimulationMode=Normal  ModelReferenceVersion=5.3
      settings: PortSchema="{\"entries\":[{\"content\":{\"sides\":[{\"content\":{\"connectorIds\":[\"In1\",\"In2\",\"In3\",\"In4\",\"In5\",\"In6\",\"In7\",\"In8\",\"In9\",\"In10\",\"In11\",\"In12\",\"In13\",\"In14\",\"In15\",\"In16\",\"In17\",\"In18\",\"In19\",\"In20\",\"In21\",\"In22\",\"In23\",\"In24\",\"In25\",\"In26\",\"In27\",\"In28\",\"In29\",\"In30\",\"In31\",\"In32\",\"In33\",\"In34\",\"In35\",\"In36\",\"In37\",\"In38\",\"In39\",\"In40\"]},\"type\":\"ConnectorPlacement.EquallySpacedRectSide\",\"uuid\":\"380f24c8-28c2-4d84-ada4-76c3689d45f6\"},{\"content\":{\"connectorIds\":[\"Out1\",\"Out2\",\"Out3\",\"Out4\",\"Out5\",\"Out6\",\"Out7\",\"Out8\",\"Out9\",\"Out10\",\"Out12\",\"Out27\",\"Out28\",\"Out11\",\"Out13\",\"Out14\",\"Out15\",\"Out16\",\"Out17\",\"Out18\",\"Out19\",\"Out20\",\"Out21\",\"Out22\",\"Out23\",\"Out24\",\"Out25\",\"Out26\"],\"side\":\"RIGHT\"},\"type\":\"ConnectorPlacement.EquallySpacedRectSide\",\"uuid\":\"ebd1e0cb-fd96-46a4-b253-2ab002a0179d\"},{\"content\":{\"side\":\"TOP\"},\"type\":\"ConnectorPlacement.EquallySpacedRectSide\",\"uuid\":\"2c6ccd3c-3f8f-4b48-bb10-6601e3a9f937\"}]},\"type\":\"ConnectorPlacement.EquallySpacedConnector\",\"uuid\":\"9fb03b06-08d2-4f18-a55b-57581e35a7b0\"}],\"packageUris\":[\"http://schema.mathworks.com/mf0/Connector/R2020b\"],\"version\":\"1.0\"}"
  Out Bus Element : Outport  PortName=Outputs  Element=LVSS_EN
  Out Bus Element1 : Outport  PortName=Outputs  Element=Fault
  Out Bus Element2 : Outport  PortName=Outputs  Element=Super_Fault
  Out Bus Element3 : Outport  PortName=Outputs  Element=Watchdog
  Out Bus Element4 : Outport  PortName=Outputs  Element=uC_State
  Out Bus Element5 : Outport  PortName=Outputs  Element=MC_EN
  Out Bus Element6 : Outport  PortName=Outputs  Element=LED
  Out Bus Element7 : Outport  PortName=Outputs  Element=CAN.Inverter_EN
  Out Bus Element8 : Outport  PortName=Outputs  Element=CAN.Fault_To_MC
  Out Bus Element9 : Outport  PortName=Outputs  Element=CAN.Inverter_DC
  Out Bus Element10 : Outport  PortName=Outputs  Element=CAN.Torque_Request
  Out Bus Element11 : Outport  PortName=Outputs  Element=CAN.BMS_Contactor_Command
  Out Bus Element12 : Outport  PortName=Outputs  Element=CAN.MC_PS_Request
  Out Bus Element13 : Outport  PortName=Outputs  Element=CAN.Batt_PS_Request
  Out Bus Element14 : Outport  PortName=Outputs  Element=CAN.HIB_EN
  Out Bus Element15 : Outport  PortName=Outputs  Element=CAN.HUDL_EN
  Out Bus Element16 : Outport  PortName=Outputs  Element=CAN.TMS_EN
  Out Bus Element17 : Outport  PortName=Outputs  Element=CAN.GUB_EN
  Out Bus Element18 : Outport  PortName=Outputs  Element=CAN.Acc_EN
  Out Bus Element19 : Outport  PortName=Outputs  Element=CAN.Batt_12V_EN
  Out Bus Element20 : Outport  PortName=Outputs  Element=CAN.Direction_Command
  Out Bus Element21 : Outport  PortName=Outputs  Element=CAN.Rolling_Counter
  Out Bus Element22 : Outport  PortName=Outputs  Element=CAN.Speed_Command
  Out Bus Element23 : Outport  PortName=Outputs  Element=CAN.Speed_Mode_EN
  Out Bus Element24 : Outport  PortName=Outputs  Element=CAN.Torque_Limit_Command
  Out Bus Element25 : Outport  PortName=Outputs  Element=LS_Self_Test_Out
  Out Bus Element27 : Outport  PortName=Outputs  Element=CAN_Self_Test
  Out Bus Element26 : Outport  PortName=Outputs  Element=MC_Self_Test
  wires:
  MCuC/26 -> Out Bus Element22/1
  MCuC/25 -> Out Bus Element21/1
  MCuC/24 -> Out Bus Element20/1
  MCuC/23 -> Out Bus Element19/1
  MCuC/22 -> Out Bus Element18/1
  MCuC/21 -> Out Bus Element17/1
  MCuC/20 -> Out Bus Element16/1
  MCuC/19 -> Out Bus Element15/1
  MCuC/18 -> Out Bus Element14/1
  MCuC/17 -> Out Bus Element13/1
  MCuC/16 -> Out Bus Element12/1
  MCuC/15 -> Out Bus Element11/1
  MCuC/14 -> Out Bus Element10/1
  MCuC/13 -> Out Bus Element9/1
  MCuC/11 -> Out Bus Element7/1
  MCuC/28 -> Out Bus Element24/1
  MCuC/27 -> Out Bus Element23/1
  MCuC/12 -> Out Bus Element8/1
  MCuC/10 -> Out Bus Element26/1
  MCuC/9 -> Out Bus Element27/1
  MCuC/8 -> Out Bus Element25/1
  MCuC/7 -> Out Bus Element6/1
  MCuC/6 -> Out Bus Element5/1
  MCuC/5 -> Out Bus Element4/1
  MCuC/4 -> Out Bus Element3/1
  MCuC/3 -> Out Bus Element2/1
  MCuC/2 -> Out Bus Element1/1
  MCuC/1 -> Out Bus Element/1
  Bus Element In40/1 -> MCuC/38
  Bus Element In39/1 -> MCuC/37
  Bus Element In38/1 -> MCuC/36
  Bus Element In37/1 -> MCuC/35
  Bus Element In36/1 -> MCuC/34
  Bus Element In35/1 -> MCuC/33
  Bus Element In34/1 -> MCuC/32
  Bus Element In33/1 -> MCuC/31
  Bus Element In32/1 -> MCuC/30
  Bus Element In31/1 -> MCuC/29
  Bus Element In30/1 -> MCuC/28
  Bus Element In29/1 -> MCuC/27
  Bus Element In28/1 -> MCuC/26
  Bus Element In27/1 -> MCuC/25
  Bus Element In26/1 -> MCuC/24
  Bus Element In25/1 -> MCuC/23
  Bus Element In24/1 -> MCuC/22
  Bus Element In23/1 -> MCuC/21
  Bus Element In22/1 -> MCuC/20
  Bus Element In21/1 -> MCuC/19
  Bus Element In20/1 -> MCuC/18
  Bus Element In19/1 -> MCuC/17
  Bus Element In18/1 -> MCuC/16
  Bus Element In17/1 -> MCuC/15
  Bus Element In16/1 -> MCuC/14
  Bus Element In15/1 -> MCuC/13
  Bus Element In14/1 -> MCuC/12
  Bus Element In13/1 -> MCuC/11
  Bus Element In12/1 -> MCuC/10
  Bus Element In11/1 -> MCuC/9
  Bus Element In10/1 -> MCuC/8
  Bus Element In9/1 -> MCuC/6
  Bus Element In8/1 -> MCuC/5
  Bus Element In7/1 -> MCuC/7
  Bus Element In6/1 -> MCuC/40
  Bus Element In5/1 -> MCuC/39
  Bus Element In4/1 -> MCuC/4
  Bus Element In3/1 -> MCuC/3
  Bus Element In2/1 -> MCuC/2
  Bus Element In1/1 -> MCuC/1

== stateflow chart TCS/Control_Logic/Torque_Display/Torque_Display ==
  state No_Display
    during:
    if Torque_Display > 0
    Torque_Display = Torque_Display - 1;
    end
  state Yes_Display
    during:
    if Brake == true && Torque_Display > 0
    Torque_Display = Torque_Display - 1;
    elseif Brake == false && Torque_Display < Torque_Command
    Torque_Display = Torque_Display + 1;
    elseif Brake == false && Torque_Display > Torque_Command
    Torque_Display = Torque_Display - 1;
    end
  (default) -> No_Display
  No_Display -> Yes_Display : [uC_State == UC_State.MC_Active]
  Yes_Display -> No_Display : [uC_State ~= UC_State.MC_Active]
  data: uC_State input; Brake input; Torque_Command input; Torque_Display output =0
